simulink model "sldemo_auto_climate_elec"  (R2024a)
settings: Solver=FixedStepAuto  StartTime=0.0  StopTime=300  MaxStep=1e-4  RelTol=1e-4  AbsTol=1e-4  EnableMultiTasking=on
undefined symbols (not defined in the file): ee
libraries: fl_lib x15, nesl_utility x10, ee_lib x8, batteryecm_lib x1, slpidlib x1, simulink x1
(part 2 of 2)

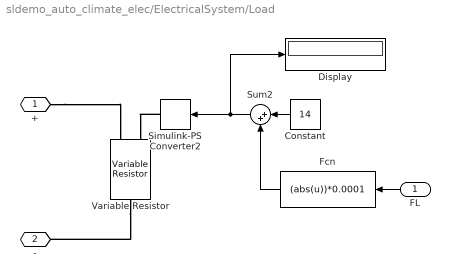
== system sldemo_auto_climate_elec/ElectricalSystem/Load ==
  FL : Inport
  Constant : Constant  Value=14
  Display : Display
  Fcn : Fcn  Expr=(abs(u))*0.0001
  Simulink-PS Converter2 : nesl_utility/Simulink-PS Converter  PhysicalDomain=network_engine_domain  SubClassName=ps_input  LeftPortType=input  RightPortType=output  PseudoPeriodic=off  Frequencies=[]  NoiseDistribution=none  NoiseParameters=[]  Unit=1  AffineConversion=off  FilteringAndDerivatives=provide  SimscapeFilterOrder=1  InputFilterTimeConstant=0.001  UdotUserProvided=0
  Sum2 : Sum  Inputs=|++  InputSameDT=on  SaturateOnIntegerOverflow=on  OutDataTypeStr=Inherit: Same as first input
  Variable Resistor : fl_lib/Electrical/Electrical Elements/Variable Resistor  Rmin=0.1 Ohm  thermalEnable=false  thermal_mass=1 J/K  i_specify=off  i_priority=None  i=0 A  i_nominal_specify=off  i_nominal_value=1  i_nominal_unit=A  v_specify=off  v_priority=None  v=0 V  v_nominal_specify=off  v_nominal_value=1  v_nominal_unit=V  T_specify=off  T_priority=None  T=300 K  T_nominal_specify=off  T_nominal_value=1  T_nominal_unit=K
  + : PMIOPort  Side=Left
  - : PMIOPort  Port=2  Side=Right
  wires:
  Sum2/1 -> Simulink-PS Converter2/1, Display/1
  Fcn/1 -> Sum2/2
  Constant/1 -> Sum2/1
  FL/1 -> Fcn/1
  connections:
  Simulink-PS Converter2/RConn1 -- Variable Resistor/LConn1
  Variable Resistor/RConn1 -- -/RConn1
  +/RConn1 -- Variable Resistor/LConn2

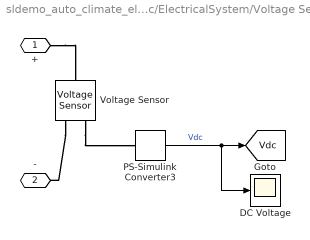
== system sldemo_auto_climate_elec/ElectricalSystem/Voltage Sensor ==
  DC Voltage : Scope
  PS-Simulink Converter3 : nesl_utility/PS-Simulink Converter  PhysicalDomain=network_engine_domain  SubClassName=ps_output  LeftPortType=input  RightPortType=output  PseudoPeriodic=off  Frequencies=[]  VectorFormat=1-D array  Unit=1  AffineConversion=off
  Voltage Sensor : fl_lib/Electrical/Electrical Sensors/Voltage Sensor
  + : PMIOPort  Side=Left
  - : PMIOPort  Port=2  Side=Right
  tag scope: Vdc=global
  wires:
  PS-Simulink Converter3/1 -> DC Voltage/1, [Vdc]  "Vdc"
  connections:
  Voltage Sensor/RConn1 -- PS-Simulink Converter3/LConn1
  Voltage Sensor/RConn2 -- -/RConn1
  +/RConn1 -- Voltage Sensor/LConn1

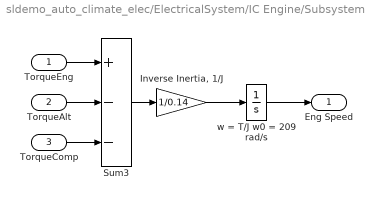
== system sldemo_auto_climate_elec/ElectricalSystem/IC Engine/Subsystem ==
  TorqueEng : Inport
  TorqueAlt : Inport  Port=2
  TorqueComp : Inport  Port=3
  "Inverse Inertia, 1/J" : Gain  Gain=1/0.14  SaturateOnIntegerOverflow=on  OutDataTypeStr=Inherit: Same as input  ParamDataTypeStr=Inherit: Same as input
  Sum3 : Sum  Inputs=+--  InputSameDT=on  SaturateOnIntegerOverflow=on  OutDataTypeStr=Inherit: Same as first input
  w = T/J w0 = 209 rad/s : Integrator  InitialCondition=209.48  ZeroCross=off
  Eng Speed : Outport  InitialOutput=0  VectorParamsAs1DForOutWhenUnconnected=off
  wires:
  w = T/J w0 = 209 rad/s/1 -> Eng Speed/1
  TorqueComp/1 -> Sum3/3
  TorqueAlt/1 -> Sum3/2
  TorqueEng/1 -> Sum3/1
  Sum3/1 -> "Inverse Inertia, 1/J"/1
  "Inverse Inertia, 1/J"/1 -> w = T/J w0 = 209 rad/s/1

== stateflow chart sldemo_auto_climate_elec/ClimateControlSystem/Temperature Control Chart ==
  state Blower [parallel]
    during:setpoint_calc();
    settings: executionOrder=1
    state Blower_off
      entry:BlowerOut=0.0;
    state Blower_on
      state Blower_1
        entry:BlowerOut=0.2;
      state Blower_2
        entry:BlowerOut=0.4;
      state Blower_3
        entry:BlowerOut=0.6;
      state Blower_4
        entry:BlowerOut=0.8;
      state Blower_5
        entry:BlowerOut=1.0;
      (default) -> Blower_1
      Blower_on -> Blower_1 [order 5] : E[~in(Blower_1) && in_temp_range(1.5,5)]
      Blower_on -> Blower_2 [order 4] : E[~in(Blower_2) && in_temp_range(7,10)]
      Blower_on -> Blower_3 [order 3] : E[~in(Blower_3) && in_temp_range(12,15)]
      Blower_on -> Blower_4 [order 2] : E[~in(Blower_4) && in_temp_range(17,20)]
      Blower_on -> Blower_5 [order 1] : E[~in(Blower_5) && in_temp_range(22,200)]
    state setpoint_calc() [function]
      (default) -> (junction 51) : {RequiredTemp = SetPTemp-IntTemp;}
      (junction 51) -> (junction 48) [order 1] : [RequiredTemp<0.0]
          | {absTempDiff = -RequiredTemp;}
      (junction 51) -> (junction 49) [order 2] : {absTempDiff = RequiredTemp;}
    state b = in_temp_range(minTemp,maxTemp) [function]
      (default) -> (junction 50) : {b = (absTempDiff>minTemp) &&  ...
          |         (absTempDiff<maxTemp);}
    (default) -> Blower_off
    Blower_off -> Blower_on : E[in_temp_range(.5,203)]
    Blower_on -> Blower_off [order 1] : E[absTempDiff>203 || absTempDiff<=0.5]
  state Heater_AC [parallel]
    settings: executionOrder=2
    state H_offAC_off
    state ACAct
    state HeaterAct
    ACAct -> H_offAC_off : E[SetPTemp-IntTemp>=-0.5]
    HeaterAct -> H_offAC_off : E[SetPTemp-IntTemp<=0.5]
    H_offAC_off -> HeaterAct [order 2] : E[SetPTemp-IntTemp>0.5]
    H_offAC_off -> ACAct [order 1] : E[SetPTemp-IntTemp<-0.5]
    (default) -> H_offAC_off
  state AirDist [parallel]
    settings: executionOrder=3
    state Feet
    state Face
    state Defrost
    (default) -> Face
    Feet -> Defrost : DistReq
    Face -> Feet : DistReq
    Defrost -> Face : DistReq
  state Recyc_Air [parallel]
    settings: executionOrder=4
    state Recyc_on
    state Recyc_off
    (default) -> Recyc_on
    Recyc_on -> Recyc_off [order 2] : RecycReq
    Recyc_off -> Recyc_on : RecycReq
    Recyc_on -> Recyc_off [order 1] : en(AirDist.Defrost)
  data: minTemp function_input double; b function_output boolean; maxTemp function_input double; ACAct output boolean; SetPTemp input double; IntTemp input double; HeaterAct output boolean; RequiredTemp output double; BlowerOut output double; absTempDiff local double
  events: DistReq input EITHER_EDGE_EVENT; RecycReq input EITHER_EDGE_EVENT; E input EITHER_EDGE_EVENT
